simulink model "struct_var_controller_robot"  (R2023b)
settings: Solver=VariableStepAuto  StartTime=0.0  StopTime=10  RelTol=1e-3
values from neighbouring files (symbols this model uses):
  A = [Alin zeros(4,1) ... (first row only)    [collaborative_class_main.m]    (also in n0_collaborative_class_main.m; svc_robot.m = [0      1       0       0)
  alfa_prime = beta_prime*A_tilde    [n0_collaborative_class_main.m]    (also in svc_robot.m = beta_prime*A)
  alfa_prime_t = beta_prime_t*F_tilde    [svc_robot.m]
  B = [0   0   0   1]'    [svc_robot.m]
  beta_prime = [p^3 3*p^2 3*p 1]    [n0_collaborative_class_main.m]    (also in svc_robot.m)
  beta_prime_t = flip(poly([p_t p_t p_t p_t]))    [svc_robot.m]
  BI = 0.02    [n0_collaborative_class_main.m]    (also in svc_robot.m)
  C = [1   0   0   0]    [svc_robot.m]
  gamma = beta3/b4    [n0_collaborative_class_main.m]    (also in svc_robot.m)
  gamma_t = beta3_t/b4_t    [svc_robot.m]
  Kv_tilde = place(A_tilde, B_tilde, p_tilde)    [collaborative_class_main.m]    (also in n0_collaborative_class_main.m)
  M = 1    [n0_collaborative_class_main.m]    (also in svc_robot.m)
  q = 1    [collaborative_class_main.m]    (also in n0_collaborative_class_main.m = 20; svc_robot.m = 20)
  r = 100    [collaborative_class_main.m]    (also in n0_collaborative_class_main.m = 0.7; svc_robot.m = 0.7)
  T = Mr_contr*Mr^-1    [n0_collaborative_class_main.m]    (also in svc_robot.m = Mr_tilde*Mr^-1)
libraries: cstblocks x1
settings Model: Creator=Kevin  LastModifiedBy=Kevin

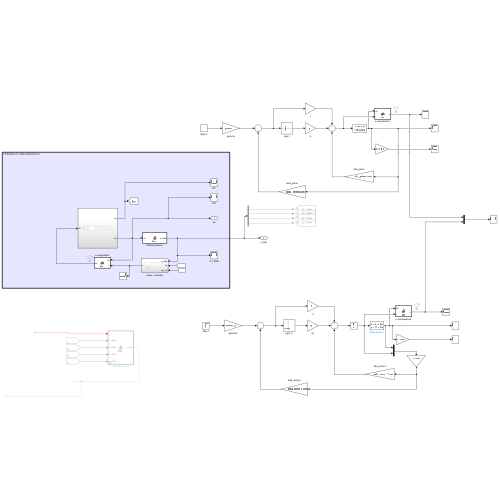
[thumbnail: Simulink's stored preview of the top-level diagram]
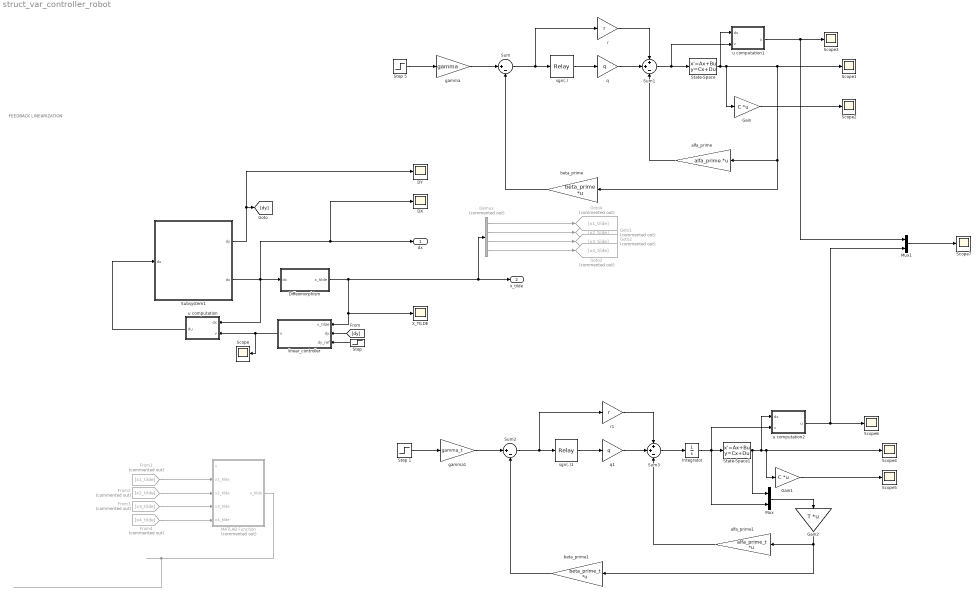
== system struct_var_controller_robot ==
  note: FEEDBACK LINEARIZATION
  DX : Scope
  DY : Scope
  Demux : Demux  Commented=on
  Diffeomorphism : MATLAB Function  TreatAsAtomicUnit=on
  From1 : From  Commented=on  GotoTag=x1_tilde
  From2 : From  Commented=on  GotoTag=x2_tilde
  From3 : From  Commented=on  GotoTag=x3_tilde
  From4 : From  Commented=on  GotoTag=x4_tilde
  Gain : Gain  Gain=C  Multiplication=Matrix(K*u) (u vector)
  Gain1 : Gain  Gain=C  Multiplication=Matrix(K*u) (u vector)
  Gain2 : Gain  Gain=T  Multiplication=Matrix(K*u) (u vector)
  Goto1 : Goto  Commented=on  GotoTag=x2_tilde
  Goto2 : Goto  Commented=on  GotoTag=x3_tilde
  Goto3 : Goto  Commented=on  GotoTag=x4_tilde
  Goto4 : Goto  Commented=on  GotoTag=x1_tilde
  Integrator : Integrator
  MATLAB Function : MATLAB Function  Commented=on  TreatAsAtomicUnit=on
  Mux : Mux  Inputs=2
  Mux1 : Mux  Inputs=2
  Scope{,1..7} (8 alike) : Scope
  State-Space : StateSpace  A=A  B=B  C=eye(4)  D=zeros(4,1)  InitialCondition=0
  State-Space1 : StateSpace  A=A  B=B  C=eye(4)  D=zeros(4,1)  InitialCondition=0
  Step : Step  Time=10  SampleTime=0
  Step 1 : Step  After=pi/4  SampleTime=0
  Step 5 : Step  After=pi/4  SampleTime=0
  Subsystem1 : Subsystem
  Sum : Sum  Inputs=|+-
  Sum1 : Sum  Inputs=++-
  Sum2 : Sum  Inputs=|+-
  Sum3 : Sum  Inputs=++-
  X_TILDE : Scope
  alfa_prime : Gain  Gain=alfa_prime  Multiplication=Matrix(K*u) (u vector)
  alfa_prime1 : Gain  Gain=alfa_prime_t  Multiplication=Matrix(K*u) (u vector)
  beta_prime : Gain  Gain=beta_prime  Multiplication=Matrix(K*u) (u vector)
  beta_prime1 : Gain  Gain=beta_prime_t  Multiplication=Matrix(K*u) (u vector)
  gamma : Gain  Gain=gamma
  gamma1 : Gain  Gain=gamma_t
  linear_controller : Subsystem
  q : Gain  Gain=q
  q1 : Gain  Gain=q
  r : Gain  Gain=r
  r1 : Gain  Gain=r
  sgn(.) : Relay  OnSwitchValue=BI/2  OffSwitchValue=-BI/2  OnOutputValue=M  OffOutputValue=-M
  sgn(.)1 : Relay  OnSwitchValue=BI/2  OffSwitchValue=-BI/2  OnOutputValue=M  OffOutputValue=-M
  u computation : MATLAB Function  TreatAsAtomicUnit=on
  u computation1 : MATLAB Function  TreatAsAtomicUnit=on
  u computation2 : MATLAB Function  TreatAsAtomicUnit=on
  dx : Outport
  x_tilde : Outport  Port=2
  wires:
  Step 5/1 -> gamma/1
  gamma/1 -> Sum/1
  Sum/1 -> r/1, sgn(.)/1
  sgn(.)/1 -> q/1
  q/1 -> Sum1/2
  r/1 -> Sum1/1
  beta_prime/1 -> Sum/2
  alfa_prime/1 -> Sum1/3
  Step/1 -> linear_controller/3(dy_ref)
  linear_controller/1(v) -> u computation/2(v), Scope/1
  Subsystem1/1(dy) -> [dy], DY/1
  u computation/1(du) -> Subsystem1/1(du)
  Diffeomorphism/1(x_tilde) -> linear_controller/1(x_tilde), X_TILDE/1, Demux/1, x_tilde/1
  [dy] -> linear_controller/2(dy)
  Subsystem1/2(dx) -> DX/1, dx/1, Diffeomorphism/1(dx), u computation/1(dx)
  Demux/1 -> Goto4/1
  Demux/2 -> Goto1/1
  Demux/3 -> Goto2/1
  Demux/4 -> Goto3/1
  From4/1 -> MATLAB Function/5(x4_tilde)
  From2/1 -> MATLAB Function/3(x2_tilde)
  ? -> MATLAB Function/1(v)
  From1/1 -> MATLAB Function/2(x1_tilde)
  MATLAB Function/1(x_tilde) -> ?
  From3/1 -> MATLAB Function/4(x3_tilde)
  State-Space/1 -> u computation1/1(dx), Gain/1, Scope1/1, beta_prime/1, alfa_prime/1
  Sum1/1 -> u computation1/2(v), State-Space/1
  Gain/1 -> Scope2/1
  u computation1/1(u) -> Mux1/1, Scope3/1
  sgn(.)1/1 -> q1/1
  Sum2/1 -> r1/1, sgn(.)1/1
  q1/1 -> Sum3/2
  State-Space1/1 -> Mux/1, u computation2/1(dx), Gain1/1, Scope4/1
  alfa_prime1/1 -> Sum3/3
  beta_prime1/1 -> Sum2/2
  Step 1/1 -> gamma1/1
  gamma1/1 -> Sum2/1
  r1/1 -> Sum3/1
  Gain1/1 -> Scope5/1
  Integrator/1 -> u computation2/2(v), State-Space1/1, Mux/2
  Gain2/1 -> beta_prime1/1, alfa_prime1/1
  Mux/1 -> Gain2/1
  Sum3/1 -> Integrator/1
  u computation2/1(u) -> Mux1/2, Scope6/1
  Mux1/1 -> Scope7/1

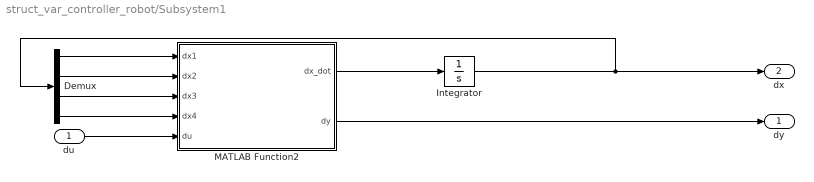
== system struct_var_controller_robot/Subsystem1 ==
  du : Inport
  Demux : Demux
  Integrator : Integrator  InitialCondition=[0;0;0;0]+1
  MATLAB Function2 : MATLAB Function  TreatAsAtomicUnit=on
  dy : Outport
  dx : Outport  Port=2
  wires:
  Integrator/1 -> Demux/1, dx/1
  du/1 -> MATLAB Function2/5(du)
  MATLAB Function2/2(dy) -> dy/1
  MATLAB Function2/1(dx_dot) -> Integrator/1
  Demux/1 -> MATLAB Function2/1(dx1)
  Demux/2 -> MATLAB Function2/2(dx2)
  Demux/3 -> MATLAB Function2/3(dx3)
  Demux/4 -> MATLAB Function2/4(dx4)

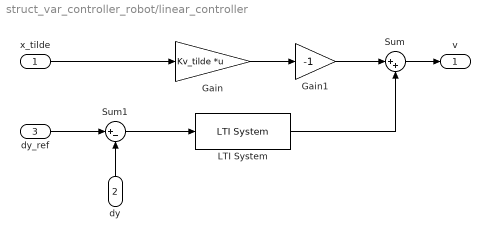
== system struct_var_controller_robot/linear_controller ==
  x_tilde : Inport
  dy : Inport  Port=2
  dy_ref : Inport  Port=3
  Gain : Gain  Gain=Kv_tilde  Multiplication=Matrix(K*u) (u vector)
  Gain1 : Gain  Gain=-1
  LTI System : cstblocks/LTI System  sys=R_v  IC=[]  PadeOrder=0
  Sum : Sum  Inputs=|++
  Sum1 : Sum  Inputs=|+-
  v : Outport
  wires:
  Gain/1 -> Gain1/1
  x_tilde/1 -> Gain/1
  Gain1/1 -> Sum/1
  Sum/1 -> v/1
  dy/1 -> Sum1/2
  dy_ref/1 -> Sum1/1
  Sum1/1 -> LTI System/1
  LTI System/1 -> Sum/2

== matlab function struct_var_controller_robot/u computation ==
  data: dx input; du output; v input
function du  = fcn(dx, v)

%v = 0;
k = 0.8;
Jm = 4e-4;
Jl= 4e-4;
Bm = 0.015;
m = 0.3;
l = 0.3;
g = 9.81;

x1_bar = 0;
x2_bar = pi/4;
x3_bar = 0;
x4_bar = m*g*l*cos(x2_bar)/k + x2_bar;
u_bar= m*g*l*cos(x2_bar);

x1 = dx(1)+x1_bar;
x2 = dx(2)+x2_bar;
x3 = dx(3)+x3_bar;
x4 = dx(4)+x4_bar;

% HARDCODED
%u = Jl*Jm/k* (   -v+k^2/Jl^2*(x4-x2)     +   m*g*l*k/Jl^2*(sin(x2)*x2-cos(x2)-sin(x2)*x4)   -    m*g*l/Jl*cos(x2)*x1^2    +   m^2*g^2*l^2/(-Jl^2)*sin(x2)*cos(x2)    +   k^2/(Jl*Jm)*(x2-x4)     +   k*Bm/(Jl*Jm)*x3);

% from MATLAB INVERSION
 u = -(Jl*Jm*((g*l*m*cos(x2)*x1^2)/Jl + v - (k*((Bm*x3)/Jm - (k*x2)/Jm + (k*x4)/Jm))/Jl + (k*((k*x2)/Jl - (k*x4)/Jl + (g*l*m*cos(x2))/Jl))/Jl - (g*l*m*sin(x2)*((k*x2)/Jl - (k*x4)/Jl + (g*l*m*cos(x2))/Jl))/Jl))/k;
du = u - u_bar;

== matlab function struct_var_controller_robot/MATLAB Function ==
  data: v input; x_tilde output; x1_tilde input; x2_tilde input; x3_tilde input; x4_tilde input
function x_tilde  = fcn(v, x1_tilde, x2_tilde, x3_tilde, x4_tilde)
    
    x1_tilde_dot= x2_tilde;
    x2_tilde_dot= x3_tilde;
    x3_tilde_dot= x4_tilde;
    x4_tilde_dot= v;
    y= x1_tilde;


x_tilde = [x1_tilde, x2_tilde, x3_tilde, x4_tilde]';

== matlab function struct_var_controller_robot/u computation1 ==
  data: dx input; u output; v input
function u  = fcn(dx, v)

%v = 0;
k = 0.8;
Jm = 4e-4;
Jl= 4e-4;
Bm = 0.015;
m = 0.3;
l = 0.3;
g = 9.81;

x1_bar = 0;
x2_bar = pi/4;
x3_bar = 0;
x4_bar = m*g*l*cos(x2_bar)/k + x2_bar;
u_bar= m*g*l*cos(x2_bar);

x1 = dx(1);
x2 = dx(2);
x3 = dx(3);
x4 = dx(4);

% HARDCODED
%u = Jl*Jm/k* (   -v+k^2/Jl^2*(x4-x2)     +   m*g*l*k/Jl^2*(sin(x2)*x2-cos(x2)-sin(x2)*x4)   -    m*g*l/Jl*cos(x2)*x1^2    +   m^2*g^2*l^2/(-Jl^2)*sin(x2)*cos(x2)    +   k^2/(Jl*Jm)*(x2-x4)     +   k*Bm/(Jl*Jm)*x3);

% from MATLAB INVERSION
 u = -(Jl*Jm*((g*l*m*cos(x2)*x1^2)/Jl + v - (k*((Bm*x3)/Jm - (k*x2)/Jm + (k*x4)/Jm))/Jl + (k*((k*x2)/Jl - (k*x4)/Jl + (g*l*m*cos(x2))/Jl))/Jl - (g*l*m*sin(x2)*((k*x2)/Jl - (k*x4)/Jl + (g*l*m*cos(x2))/Jl))/Jl))/k;

== matlab function struct_var_controller_robot/Subsystem1/MATLAB Function2 ==
  data: dx1 input; dx2 input; dx3 input; dx4 input; du input; dx_dot output; dy output
function [dx_dot, dy]  = fcn(dx1,dx2,dx3,dx4, du)

k = 0.8;
Jm = 4e-4;
Jl= 4e-4;
Bm = 0.015;
Bl = 0;
m = 0.3;
l = 0.3;
g = 9.81;
x1_bar = 0;
x2_bar = pi/4;
x3_bar = 0;
x4_bar = m*g*l*cos(x2_bar)/k + x2_bar;
u_bar= m*g*l*cos(x2_bar);


dx1_dot = -k/Jl*(dx2+x2_bar)-m*g*l/Jl*(cos(dx2+x2_bar))+k/Jl*(dx4+x4_bar);
dx2_dot = dx1+x1_bar;
dx3_dot = k/Jm*(dx2+x2_bar)-Bm/Jm*(dx3+x3_bar)-k/Jm*(dx4+x4_bar)+1/Jm*(du+u_bar);
dx4_dot = dx3+x3_bar;
dy = pi/4 - (dx2+x2_bar);

dx_dot = zeros(1,4);
dx_dot(1) = dx1_dot;
dx_dot(2) = dx2_dot;
dx_dot(3) = dx3_dot;
dx_dot(4) = dx4_dot;

== matlab function struct_var_controller_robot/Diffeomorphism ==
  data: dx input; x_tilde output
function x_tilde  = fcn(dx)

dx1 = dx(1);
dx2 = dx(2);
dx3 = dx(3);
dx4 = dx(4);
k = 0.8;
Jm = 4e-4;
Jl= 4e-4;
Bm = 0.015;
Bl = 0;
m = 0.3;
l = 0.3;
g = 9.81;

x1_tilde = -dx2;
x2_tilde = -dx1;
x3_tilde = (k*(pi/4 + dx2))/Jl - (k*(dx4 + sqrt(2)/2*m*g*l/k+pi/4))/Jl + (g*l*m*cos(pi/4 + dx2))/Jl;
x4_tilde = (k*dx1)/Jl - (k*dx3)/Jl - (g*l*m*sin(pi/4 + dx2)*dx1)/Jl;

x_tilde = zeros(length(dx),1);
x_tilde(1) = x1_tilde;
x_tilde(2) = x2_tilde;
x_tilde(3) = x3_tilde;
x_tilde(4) = x4_tilde;

== matlab function struct_var_controller_robot/u computation2 ==
  data: dx input; u output; v input
function u  = fcn(dx, v)

%v = 0;
k = 0.8;
Jm = 4e-4;
Jl= 4e-4;
Bm = 0.015;
m = 0.3;
l = 0.3;
g = 9.81;

x1_bar = 0;
x2_bar = pi/4;
x3_bar = 0;
x4_bar = m*g*l*cos(x2_bar)/k + x2_bar;
u_bar= m*g*l*cos(x2_bar);

x1 = dx(1);
x2 = dx(2);
x3 = dx(3);
x4 = dx(4);

% HARDCODED
%u = Jl*Jm/k* (   -v+k^2/Jl^2*(x4-x2)     +   m*g*l*k/Jl^2*(sin(x2)*x2-cos(x2)-sin(x2)*x4)   -    m*g*l/Jl*cos(x2)*x1^2    +   m^2*g^2*l^2/(-Jl^2)*sin(x2)*cos(x2)    +   k^2/(Jl*Jm)*(x2-x4)     +   k*Bm/(Jl*Jm)*x3);

% from MATLAB INVERSION
 u = -(Jl*Jm*((g*l*m*cos(x2)*x1^2)/Jl + v - (k*((Bm*x3)/Jm - (k*x2)/Jm + (k*x4)/Jm))/Jl + (k*((k*x2)/Jl - (k*x4)/Jl + (g*l*m*cos(x2))/Jl))/Jl - (g*l*m*sin(x2)*((k*x2)/Jl - (k*x4)/Jl + (g*l*m*cos(x2))/Jl))/Jl))/k;
